simulink model "s0509_Ly_bang"  (R2019b)
settings: Solver=ode1  StartTime=0.0  StopTime=100  FixedStep=dt  RelTol=1e-3
values from neighbouring files (symbols this model uses):
  dt = 1e-4    (= 0.0001)    [m0303_init.m]    (also in m0310_init.m = mean(diff(log.time)); m0312_init.m; m0314_init.m = 0.002; m0318_init.m = 0.0002)
  PARAMS =     [s0310_main.mat]
settings Model: Creator=paolo  LastModifiedBy=alessandro
settings DebuggingCC: AlgebraicLoopMsg=none  SFMachineParentedDataDiag=error  ArithmeticOperatorsInVariantConditions=warning
settings SFSimCC: CustomCodeUndefinedFunction=UseInterfaceOnly
settings CodeAppCC: StateflowObjectComments=on

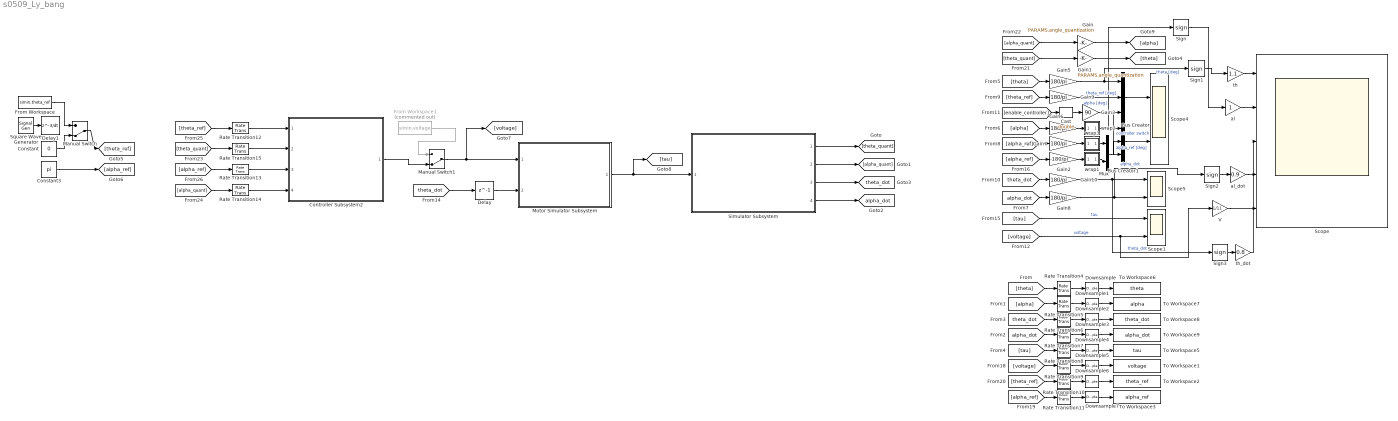
== system s0509_Ly_bang ==
  Bus Creator : BusCreator  Inputs=3
  Bus Creator1 : BusCreator  Inputs=3
  Cast : DataTypeConversion  OutDataTypeStr=double
  Constant : Constant  Value=0
  Constant3 : Constant  Value=pi
  Controller Subsystem2 : Subsystem  ReferencedSubsystem=s0326_Bad_Lyapunov  K_th=0.015  K_th_dot=0.001  K_al=0.015  K_al_dot=0
  Delay : Delay  DelayLength=1  InitialCondition=PARAMS.th_dot_0
  Delay1 : Delay  DelayLength=3/dt
  Downsample{,1..7} (8 alike) : DownSample  N=ceil((2e-3)/dt)  RateOptions=Allow multirate processing
  From Workspace : FromWorkspace  VariableName=simin.theta_ref  SampleTime=0
  From Workspace1 : FromWorkspace  Commented=on  VariableName=simin.voltage  SampleTime=0
  Gain : Gain  Gain=PARAMS.angle_quantization
  Gain1 : Gain  Gain=PARAMS.angle_quantization
  Gain{5..10} (6 alike) : Gain  Gain=180/pi
  Gain2 : Gain  Gain=-180/pi
  Gain3 : Gain  Gain=90
  Manual Switch : ManualSwitch  CurrentSetting=0
  Manual Switch1 : ManualSwitch  CurrentSetting=0
  Motor Simulator Subsystem : Subsystem  ReferencedSubsystem=s0303_motor_simulator  omega_0=PARAMS.th_dot_0  i_0=0
  Mux : Mux  Inputs=2
  Rate Transition{4..11} (8 alike) : RateTransition  OutPortSampleTime=dt
  Rate Transition{12..15} (4 alike) : RateTransition  OutPortSampleTime=dt_control
  Scope : Scope  NumInputPorts=5
  Scope1 : Scope  NumInputPorts=2
  Scope4 : Scope  NumInputPorts=2
  Scope5 : Scope  NumInputPorts=2
  Sign{,1..3} (4 alike) : Signum
  Simulator Subsystem : Subsystem  ReferencedSubsystem=s0405_mechanical_simulator  th_0=PARAMS.th_0  al_0=PARAMS.al_0-pi*179.9/180  th_dot_0=PARAMS.th_dot_0  al_dot_0=PARAMS.al_dot_0
  Square Wave Generator : SignalGenerator  WaveForm=square  Amplitude=pi/6  Frequency=0.2  Units=rad/sec
  To Workspace1 : ToWorkspace  VariableName=voltage  SaveFormat=Timeseries  SampleTime=-1
  To Workspace2 : ToWorkspace  VariableName=theta_ref  SaveFormat=Timeseries  SampleTime=-1
  To Workspace3 : ToWorkspace  VariableName=alpha_ref  SaveFormat=Timeseries  SampleTime=-1
  To Workspace5 : ToWorkspace  VariableName=tau  SaveFormat=Timeseries  SampleTime=-1
  To Workspace6 : ToWorkspace  VariableName=theta  SaveFormat=Timeseries  SampleTime=-1
  To Workspace7 : ToWorkspace  VariableName=alpha  SaveFormat=Timeseries  SampleTime=-1
  To Workspace8 : ToWorkspace  VariableName=theta_dot  SaveFormat=Timeseries  SampleTime=-1
  To Workspace9 : ToWorkspace  VariableName=alpha_dot  SaveFormat=Timeseries  SampleTime=-1
  V : Gain  Gain=1/11
  al : Gain
  al_dot : Gain  Gain=0.9
  th : Gain  Gain=1.1
  th_dot : Gain  Gain=0.8
  wrap1 : MATLAB Function  TreatAsAtomicUnit=on
  wrap2 : MATLAB Function  TreatAsAtomicUnit=on
  wrap3 : MATLAB Function  TreatAsAtomicUnit=on
  tag scope: alpha_dot=global, theta_dot=global
  wires:
  Simulator Subsystem/1 -> [theta_quant]
  Simulator Subsystem/2 -> [alpha_quant]
  Simulator Subsystem/4 -> [alpha_dot]
  Simulator Subsystem/3 -> [theta_dot]
  Motor Simulator Subsystem/1 -> Simulator Subsystem/1, [tau]
  Bus Creator/1 -> Scope4/1
  [alpha_ref] -> Gain7/1
  [theta] -> Gain5/1
  [alpha] -> Gain6/1
  Gain8/1 -> Sign2/1, Scope5/2  "alpha_dot"
  Bus Creator1/1 -> Scope4/2
  [theta_dot] -> Gain10/1
  [alpha_dot] -> Gain8/1
  Gain10/1 -> Sign3/1, Scope5/1  "theta_dot"
  [theta_ref] -> Gain9/1
  [theta_dot] -> Delay/1
  [voltage] -> V/1, Scope1/2  "voltage"
  Constant3/1 -> [alpha_ref]
  [tau] -> Scope1/1  "tau"
  Delay/1 -> Motor Simulator Subsystem/2
  [theta] -> Rate Transition4/1
  [alpha] -> Rate Transition5/1
  [theta_dot] -> Rate Transition6/1
  [alpha_dot] -> Rate Transition7/1
  [tau] -> Rate Transition8/1
  [voltage] -> Rate Transition9/1
  [theta_ref] -> Rate Transition10/1
  [alpha_ref] -> Rate Transition11/1
  Downsample7/1 -> To Workspace3/1
  Downsample6/1 -> To Workspace2/1
  Downsample5/1 -> To Workspace1/1
  Downsample4/1 -> To Workspace5/1
  Downsample3/1 -> To Workspace9/1
  Downsample2/1 -> To Workspace8/1
  Downsample1/1 -> To Workspace7/1
  Downsample/1 -> To Workspace6/1
  Rate Transition4/1 -> Downsample/1
  Rate Transition5/1 -> Downsample1/1
  Rate Transition6/1 -> Downsample2/1
  Rate Transition7/1 -> Downsample3/1
  Rate Transition8/1 -> Downsample4/1
  Rate Transition9/1 -> Downsample5/1
  Rate Transition10/1 -> Downsample6/1
  Rate Transition11/1 -> Downsample7/1
  Gain9/1 -> Bus Creator/2  "theta_ref [deg]"
  wrap2/1(y) -> Sign/1, Bus Creator1/1  "alpha [deg]"
  Gain6/1 -> wrap2/1(u)
  Gain7/1 -> wrap3/1(u)
  Gain5/1 -> Sign1/1, Bus Creator/1  "theta [deg]"
  [alpha_quant] -> Gain/1
  Gain/1 -> [alpha]
  Gain1/1 -> [theta]
  [theta_quant] -> Gain1/1
  [alpha_quant] -> Rate Transition14/1
  [alpha_ref] -> Rate Transition13/1
  [theta_quant] -> Rate Transition15/1
  Rate Transition15/1 -> Controller Subsystem2/2
  [theta_ref] -> Rate Transition12/1
  Rate Transition13/1 -> Controller Subsystem2/3
  Rate Transition12/1 -> Controller Subsystem2/1
  Rate Transition14/1 -> Controller Subsystem2/4
  wrap3/1(y) -> Mux/1
  Mux/1 -> Bus Creator1/2  "alpha_ref [deg]"
  Gain2/1 -> wrap1/1(u)
  [alpha_ref] -> Gain2/1
  wrap1/1(y) -> Mux/2
  Square Wave Generator/1 -> Delay1/1
  Manual Switch/1 -> [theta_ref]
  From Workspace/1 -> Manual Switch/1
  Constant/1 -> Manual Switch/2
  [enable_controller] -> Cast/1
  Gain3/1 -> Bus Creator1/3, Bus Creator/3  "controller switch"
  Cast/1 -> Gain3/1
  Manual Switch1/1 -> [voltage], Motor Simulator Subsystem/1
  From Workspace1/1 -> Manual Switch1/1
  Controller Subsystem2/1 -> Manual Switch1/2
  Sign/1 -> al/1
  Sign1/1 -> th/1
  Sign2/1 -> al_dot/1
  Sign3/1 -> th_dot/1
  al/1 -> Scope/2
  th/1 -> Scope/1
  al_dot/1 -> Scope/4
  th_dot/1 -> Scope/3
  V/1 -> Scope/5

== matlab function s0509_Ly_bang/wrap2 ==
  data: u input; y output
function y = wrap(u)
stop_condition = false;
y = u;
while ~stop_condition
    if y > 270
        y = y - 360;
    elseif y < -270
        y = y + 360;
    else
        stop_condition = true;
    end
end

== matlab function s0509_Ly_bang/wrap3 ==
  data: u input; y output
function y = wrap(u)
stop_condition = false;
y = u;
while ~stop_condition
    if y > 270
        y = y - 360;
    elseif y < -270
        y = y + 360;
    else
        stop_condition = true;
    end
end

== matlab function s0509_Ly_bang/wrap1 ==
  data: u input; y output
function y = wrap(u)
stop_condition = false;
y = u;
while ~stop_condition
    if y > 270
        y = y - 360;
    elseif y < -270
        y = y + 360;
    else
        stop_condition = true;
    end
end
